simulink library "spikertlib"  (R2024b)
settings: Solver=FixedStepAuto  StartTime=0.0  StopTime=10.0  RelTol=1e-3
libraries: simulink x1, $bdroot x1
settings Model: Creator=ymatsuur  LastModifiedBy=yokano
settings OptimizationCC: DefaultParameterBehavior=Inlined  EnhancedBackFolding=on  PassReuseOutputArgsAs=Individual arguments  ZeroExternalMemoryAtStartup=off  ZeroInternalMemoryAtStartup=off  OptimizeBlockOrder=speed  DifferentSizesBufferReuse=on  OptimizationCustomize=off  EfficientTunableParamExpr=on
settings DebuggingCC: ParameterTunabilityLossMsg=error
settings SFSimCC: MATLABDynamicMemAlloc=off
settings RTWCC: Description=Embedded Coder  SystemTargetFile=ert.tlc  GenCodeOnly=on  TemplateMakefile=ert_default_tmf  GPUComputeCapability=3.5
settings CodeAppCC: ForceParamTrailComments=on  IgnoreCustomStorageClasses=off  OperatorAnnotations=on  SimulinkDataObjDesc=on  SFDataObjDesc=on  InsertBlockDesc=on
settings ERTTargetCC: TargetLangStandard=C99 (ISO)  GenerateSampleERTMain=on  IncludeMdlTerminateFcn=off  ERTCustomFileTemplate=addspikertmain.tlc  ERTFilePackagingFormat=Compact

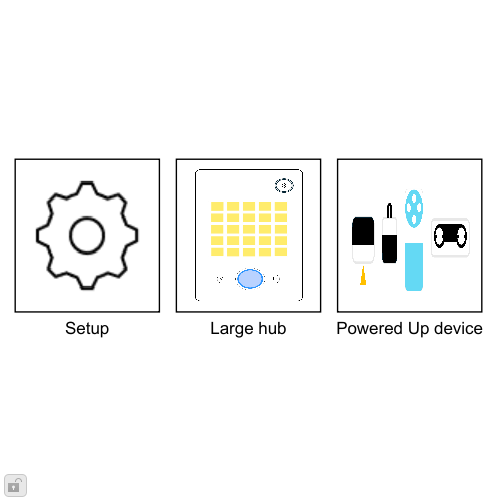
[thumbnail: Simulink's stored preview of the top-level diagram]
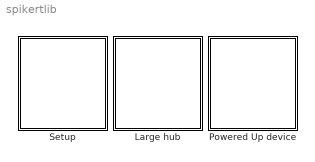
== system spikertlib ==
  Large hub : Subsystem
      mask Display: image('sphub.png'); % 変更するには、ツールストリップの [イメージの編集] を使用してください。
  Powered Up device : Subsystem
      mask Display: image('sppup.png'); % 変更するには、ツールストリップの [イメージの編集] を使用してください。
  Setup : Subsystem
      mask Display: image('spmodelsetup.png');

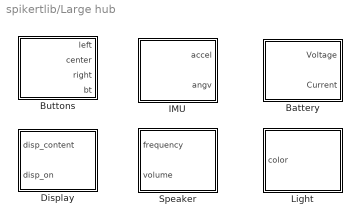
== system spikertlib/Large hub ==
  Battery : Subsystem  mask(Battery){}
      mask help: Retrieve the battery voltage [mV] and the battery current[mA].
      mask Display: image('spbattery.png');
  Buttons : Subsystem  mask(Buttons){}
      mask help: Checks which buttons (left, center, right, bluetooth) are currently pressed. (0=Not pressed, 1=Pressed)
      mask Display: image('spbutton.png');
  Display : Subsystem  mask(Pup device){Mode=Numeric, UpOrientation=RIGHT}
      mask prompts: UpOrientation "Upside orientation"
      mask help:
      | [Numeric]
      | Displays a number in the range -99 to 99. A minus sign (-) is shown as a faint dot in the center of the display. Upside orientation is set to TOP, LEFT, RIGHT, BOTTOM.
      |
      | [Character]
      | Display one character at a time if dispOn is greater than 0. Character input must be string type. Upside orientation is set to TOP, LEFT, RIGHT, BOTTOM.
      |
      | [Matrix]
      | Displays brightness matrix of Mux array in the range of 0-100. Upside orientation is set to TOP, LEFT, RIGHT, BOTTOM.
      mask TypeOptions Mode: Numeric | Character | Matrix
      mask TypeOptions UpOrientation: TOP | LEFT | RIGHT | BOTTOM
      mask DialogControl ParameterGroupVar Prompt: パラメーター
      mask Display: image('spdisplay.png');
  IMU : Subsystem  mask(Imu){}
      mask help:
      | Get the acceleration and angular velocity by the IMU.
      | accel: The vector signal which contains x, y, z axes of the acceleration [mm/s^2].
      | angv: The vector signal which contains x, y, z axes of the angular velocity [deg/sec].
      mask Display: image('spimu.png');
  Light : Subsystem  mask(Light){}
      mask help: Turn the light on with specified color (0=White, 1=Red, 2=Orange, 3=Yellow, 4=Green, 5=Blue, 6=Indigo, 7=Purple, Others=Off).
      mask Display: image('splight.png');
  Speaker : Subsystem  mask(Speaker){}
      mask help:
      | Set the volume level of the speaker and play a tone.
      | volume range 0-100[%], and frequency range 0-24000[Hz].
      mask Display: image('spspeaker.png');

== system spikertlib/Powered Up device ==
  PortA In : Subsystem  mask(Pup device){PortID=A, SensorType=Force, SensorMode=Reflection, LightOn=on}
      mask prompts: PortID "Port"; SensorType "Sensor type"; SensorMode "Sensor mode"; LightOn "Light on"
      mask help:
      | [Force sensor]
      | Force sensor detects the force [N] (range: about 0-10).
      |
      | [Color sensor]
      | Color sensor detect the reflection, ambient light, or color (HSV).
      | Reflection: Get the percentage of how much a surface reflects the light emitted by the sensor. [%] (100= white, 50= gray, 01=black, 00=No surface in front of the sensor.)
      | Ambient: Get the ambient light intensity (range: 0=dark, 100=bright)
      | Color: Get the color of surface. (0=Others, 1=Red, 2=Orange, 3=Yellow, 4=Green, 5=Blue, 6=Indigo, 7=Violet)
      |
      | [Ultrasonic sensor]
      | Get the distance [mm] in front of the ultrasonic sensor. (range: 0-2000, 2000 if no obstacles in front of the sensor.)
      |
      | [Motor]
      | Get the angle[deg] angle velocity [deg/s] of the motor.
      | !! Need Motor block in the same model for initialization. !!
      |
      | [None]
      | No sensor exsists.
      mask TypeOptions PortID: A | B | C | D | E | F
      mask Callback PortID:
      | outportHandle = get_param([gcb, '/Out1'], 'PortHandles');
      |     lineHandle = get_param(outportHandle.Inport, 'Line');
      |     set_param(lineHandle, 'Name', get_param(gcb, 'SensorType') +"_"+ get_param(gcb, 'PortID'));
      mask TypeOptions SensorType: Force | Color | Ultrasonic | Motor | None
      mask Callback SensorType:
      | if get_param(gcb, 'SensorType') == "Force"
      |         set_param(gcb, 'MaskVisibilities', {'on', 'on', 'off', 'off'});
      |     elseif get_param(gcb, 'SensorType') == "Color"
      |         set_param(gcb, 'MaskVisibilities', {'on', 'on', 'on', 'on'});
      |     elseif get_param(gcb, 'SensorType') == "Ultrasonic"
      |         set_param(gcb, 'MaskVisibilities', {'on', 'on', 'off', 'on'});
      |     else
      |         set_param(gcb, 'MaskVisibilities', {'on', 'on', 'off', 'off'});
      |     end
      | 
      |     outportHandle = get_param([gcb, '/Out1'], 'PortHandles');
      |     lineHandle = get_param(outportHandle.Inport, 'Line');
      |     set_param(lineHandle, 'Name', get_param(gcb, 'SensorType') +"_"+ get_param(gcb, 'PortID'));
      mask TypeOptions SensorMode: Reflection | Ambient | Color
      mask DialogControl ParameterGroupVar Prompt: パラメーター
      mask Display:
      | switch get_param(gcb, 'SensorType')
      |     case "Force"
      |         image('spforcesensor.png');
      |     case "Color"
      |         image('spcolorsensor.png');
      |     case "Ultrasonic"
      |         image('spultrasonicsensor.png');
      |     case "Motor"
      |         image('spmotor.png');
      |     case 5
      |         disp("");
      | end
      | 
      | color('red');
      | switch get_param(gcb, 'PortID')
      |     case "A"
      |         text(0.7, 0.1, 'Port: A');
      |     case "B"
      |         text(0.7, 0.1, 'Port: B');
      |     case "C"
      |         text(0.7, 0.1, 'Port: C');
      |     case "D"
      |         text(0.7, 0.1, 'Port: D');
      |     case "E"
      |         text(0.7, 0.1, 'Port: E');
      |     case "F"
      |         text(0.7, 0.1, 'Port: F');
      | end
  PortA Out : Subsystem  mask(Pup device){PortID=A, Mode=Set the speed of rotation [deg/s], EncorderReset=No reset, Direction=Clockwise}
      mask prompts: PortID "Port"; Mode "Motor mode"; EncorderReset "Encorder"
      mask help:
      | [Motor mode]
      | Set the speed of rotation[deg/s]: Control the motor speed at the specified value.
      | Set the power of the motor[%]: Set the motor voltage.
      | Stop: Stop the motor. But, the encoder is active and the value can be used.
      |
      | [Encorder]
      | No reset: Initial encorder value is set to an absolute angle.
      | Reset: Initial encorder value is set to 0.
      mask TypeOptions PortID: A | B | C | D | E | F
      mask Callback PortID:
      | outportHandle = get_param([gcb, '/In1'], 'PortHandles');
      |     lineHandle = get_param(outportHandle.Outport, 'Line');
      | 
      |     if get_param(gcb, 'Mode') == "None"
      |         set_param(gcb, 'MaskVisibilities', {'on', 'on', 'off', 'off'});
      |         set_param(lineHandle, 'Name', "Motor_"+ get_param(gcb, 'PortID'));
      |     else
      |         set_param(gcb, 'MaskVisibilities', {'on', 'on', 'on', 'on'});
      |         set_param(lineHandle, 'Name', "None_"+ get_param(gcb, 'PortID'));
      |     end
      mask Callback Mode:
      | outportHandle = get_param([gcb, '/In1'], 'PortHandles');
      |     lineHandle = get_param(outportHandle.Outport, 'Line');
      | 
      |     if get_param(gcb, 'Mode') == "None"
      |         set_param(gcb, 'MaskVisibilities', {'on', 'on', 'off', 'off'});
      |         set_param(lineHandle, 'Name', "Motor_"+ get_param(gcb, 'PortID'));
      |     else
      |         set_param(gcb, 'MaskVisibilities', {'on', 'on', 'on', 'on'});
      |         set_param(lineHandle, 'Name', "None_"+ get_param(gcb, 'PortID'));
      |     end
      mask TypeOptions EncorderReset: No reset | Reset
      mask TypeOptions Direction: Clockwise | Couter-clockwise
      mask DialogControl ParameterGroupVar Prompt: パラメーター
      mask Display:
      | if get_param(gcb, 'Mode') == "None"
      | 
      | else
      |     image('spmotor.png');
      | end
      | 
      | 
      | color('red');
      | switch get_param(gcb, 'PortID')
      |     case "A"
      |         text(0.7, 0.1, 'Port: A');
      |     case "B"
      |         text(0.7, 0.1, 'Port: B');
      |     case "C"
      |         text(0.7, 0.1, 'Port: C');
      |     case "D"
      |         text(0.7, 0.1, 'Port: D');
      |     case "E"
      |         text(0.7, 0.1, 'Port: E');
      |     case "F"
      |         text(0.7, 0.1, 'Port: F');
      | end

== system spikertlib/Setup ==
  Callback Button : CustomCallbackButton  Description=Generate and build code. write executable to SPIKE  Configuration="{\"components\":[{\"name\":\"BackgroundImageComponent\",\"settings\":{\"image\":{\"size\":[0,0],\"src\":\"default\",\"srcOrientation\":\"Right\"},\"position\":[0,0,1,1]}},{\"name\":\"ButtonStateComponent\",\"settings\":{\"buttonType\":\"momentary\",\"clickFcn\":\"controlsetupspikert_callback;\\ncopyspikert(2)\\ncopyspikert(3)\",\"latched\":false,\"offValue\":null,\"onValue\":1,\"position\":[0,0,1,1],\"pressDelay\":\"500\",\"pressFcn\":\"\",\"repeatInterval\":\"0\",\"states\":[{\"horizontalAlignment\":\"center\",\"image\":{\"position\":[0,0,1,1],\"size\":[1,1],\"src\":\"default\",\"srcOrientation\":\"Right\"},\"label\":{\"color\":[1,1,1],\"icon\":{\"size\":[0,0],\"src\":\"default\",\"srcOrientation\":\"Right\"},\"iconOffset\":0,\"iconPlacement\":\"left\",\"opacity\":1,\"show\":true,\"text\":{\"content\":\"Build & Write\",\"font\":\"Helvetica\"}},\"labelOffset\":[0,0],\"verticalAlignment\":\"middle\"},{\"horizontalAlignment\":\"center\",\"image\":{\"position\":[0,0,1,1],\"size\":[1,1],\"src\":\"default\",\"srcOrientation\":\"Right\"},\"label\":{\"color\":[0.01176470588,0.01176470588,0.01176470588,1],\"icon\":{\"size\":[0,0],\"src\":\"default\",\"srcOrientation\":\"Right\"},\"iconOffset\":0,\"iconPlacement\":\"left\",\"opacity\":1,\"show\":true,\"text\":{\"content\":\"Build & Write\",\"font\":\"Helvetica\"}},\"labelOffset\":[0,0],\"verticalAlignment\":\"middle\"},{\"horizontalAlignment\":\"center\",\"image\":{\"position\":[0,0,1,1],\"size\":[1,1],\"src\":\"default\",\"srcOrientation\":\"Right\"},\"label\":{\"color\":[0.01176470588,0.01176470588,0.01176470588,1],\"icon\":{\"size\":[0,0],\"src\":\"default\",\"srcOrientation\":\"Right\"},\"iconOffset\":0,\"iconPlacement\":\"left\",\"opacity\":1,\"show\":true,\"text\":{\"content\":\"Build & Write\",\"font\":\"Helvetica\"}},\"labelOffset\":[0,0],\"verticalAlignment\":\"middle\"},{\"horizontalAlignment\":\"center\",\"image\":{\"position\":[0,0,1,1],\"size\":[1,1],\"src\":\"default\",\"srcOrientation\":\"Right\"},\"label\":{\"color\":[0.01176470588,0.01176470588,0.01176470588,1],\"icon\":{\"size\":[0,0],\"src\":\"default\",\"srcOrientation\":\"Right\"},\"iconOffset\":0,\"iconPlacement\":\"left\",\"opacity\":1,\"show\":true,\"text\":{\"content\":\"Build & Write\",\"font\":\"Helvetica\"}},\"labelOffset\":[0,0],\"verticalAlignment\":\"middle\"}]}},{\"name\":\"ForegroundImageComponent\",\"settings\":{\"image\":{\"size\":[0,0],\"src\":\"default\",\"srcOrientation\":\"Right\"},\"isForeground\":1,\"position\":[0,0,1,1]}}],\"settings\":{\"BindingType\":\"standalone\",\"backgroundColor\":[244,244,244,1],\"backgroundOffset\":0.2,\"backgroundOpacity\":1,\"fixedAspectRatio\":\"off\",\"foregroundColor\":[0.01176470588,0.01176470588,0.01176470588,1],\"migratedFromLegacy\":true,\"useBackgroundColor\":true,\"variant\":\"callback\",\"version\":\"R2023a\"},\"type\":\"Button\"}"  CustomBackgroundColor="{\"color\":[0.8509803921568627,0.3254901960784314,0.09803921568627451],\"show\":true}"
  Callback Button1 : CustomCallbackButton  Description=Generate and build code. write executable to SPIKE  Configuration="{\"components\":[{\"name\":\"BackgroundImageComponent\",\"settings\":{\"image\":{\"size\":[0,0],\"src\":\"default\",\"srcOrientation\":\"Right\"},\"position\":[0,0,1,1]}},{\"name\":\"ButtonStateComponent\",\"settings\":{\"buttonType\":\"momentary\",\"clickFcn\":\"copyspikert(4)\",\"latched\":false,\"offValue\":null,\"onValue\":1,\"position\":[0,0,1,1],\"pressDelay\":\"500\",\"pressFcn\":\"\",\"repeatInterval\":\"0\",\"states\":[{\"horizontalAlignment\":\"center\",\"image\":{\"position\":[0,0,1,1],\"size\":[1,1],\"src\":\"default\",\"srcOrientation\":\"Right\"},\"label\":{\"color\":[1,1,1],\"icon\":{\"size\":[0,0],\"src\":\"default\",\"srcOrientation\":\"Right\"},\"iconOffset\":0,\"iconPlacement\":\"left\",\"opacity\":1,\"show\":true,\"text\":{\"content\":\"Restore original firmware\",\"font\":\"Helvetica\"}},\"labelOffset\":[0,0],\"verticalAlignment\":\"middle\"},{\"horizontalAlignment\":\"center\",\"image\":{\"position\":[0,0,1,1],\"size\":[1,1],\"src\":\"default\",\"srcOrientation\":\"Right\"},\"label\":{\"color\":[0.01176470588,0.01176470588,0.01176470588,1],\"icon\":{\"size\":[0,0],\"src\":\"default\",\"srcOrientation\":\"Right\"},\"iconOffset\":0,\"iconPlacement\":\"left\",\"opacity\":1,\"show\":true,\"text\":{\"content\":\"Restore original firmware\",\"font\":\"Helvetica\"}},\"labelOffset\":[0,0],\"verticalAlignment\":\"middle\"},{\"horizontalAlignment\":\"center\",\"image\":{\"position\":[0,0,1,1],\"size\":[1,1],\"src\":\"default\",\"srcOrientation\":\"Right\"},\"label\":{\"color\":[0.01176470588,0.01176470588,0.01176470588,1],\"icon\":{\"size\":[0,0],\"src\":\"default\",\"srcOrientation\":\"Right\"},\"iconOffset\":0,\"iconPlacement\":\"left\",\"opacity\":1,\"show\":true,\"text\":{\"content\":\"Restore original firmware\",\"font\":\"Helvetica\"}},\"labelOffset\":[0,0],\"verticalAlignment\":\"middle\"},{\"horizontalAlignment\":\"center\",\"image\":{\"position\":[0,0,1,1],\"size\":[1,1],\"src\":\"default\",\"srcOrientation\":\"Right\"},\"label\":{\"color\":[0.01176470588,0.01176470588,0.01176470588,1],\"icon\":{\"size\":[0,0],\"src\":\"default\",\"srcOrientation\":\"Right\"},\"iconOffset\":0,\"iconPlacement\":\"left\",\"opacity\":1,\"show\":true,\"text\":{\"content\":\"Restore original firmware\",\"font\":\"Helvetica\"}},\"labelOffset\":[0,0],\"verticalAlignment\":\"middle\"}]}},{\"name\":\"ForegroundImageComponent\",\"settings\":{\"image\":{\"size\":[0,0],\"src\":\"default\",\"srcOrientation\":\"Right\"},\"isForeground\":1,\"position\":[0,0,1,1]}}],\"settings\":{\"BindingType\":\"standalone\",\"backgroundColor\":[244,244,244,1],\"backgroundOffset\":0.2,\"backgroundOpacity\":1,\"fixedAspectRatio\":\"off\",\"foregroundColor\":[0.01176470588,0.01176470588,0.01176470588,1],\"migratedFromLegacy\":true,\"useBackgroundColor\":true,\"variant\":\"callback\",\"version\":\"R2023a\"},\"type\":\"Button\"}"  CustomBackgroundColor="{\"color\":[0,0.4470588235294118,0.7411764705882353],\"show\":true}"

== system spikertlib/Large hub/Battery ==
  Battery : S-Function  FunctionName=Battery  SFunctionDeploymentMode=off  EnableBusSupport=off  mask(Legacy Function){SFunctionSpec=Battery(double y1, double y2), ShowSpec=on}
      mask prompts: ShowSpec "表示関数の仕様"
      mask help:
      | このブロックは、以下の Legacy Code Tool の定義で指定されたレガシ関数を呼び出すことができます:
      | def.SFunctionName = 'Battery';
      | def.OutputFcnSpec = 'Battery(double y1, double y2)';
      | def.HeaderFiles = {'sfunspikert.h'};
      | def.SourceFiles = {'sfunspikert.c'};
      | def.IncPaths = {'C:\class\coursefiles\SPIKE_Dev\libblocks'};
      mask Help: <p>このブロックは、Legacy Code Tool で自動的に生成されました。このツールと呼び出しの詳細は、ヘルプを参照してください。<a href="matlab:legacy_code('help')"> legacy_code('help')</a>.</p>
      mask Callback ShowSpec:
      | if strcmp(get_param(gcbh, 'ShowSpec'), 'on')
      |   set_param(gcbh, 'MaskDisplay', sprintf('fprintf(''%s'');', get_param(gcbh, 'SFunctionSpec')));
      | else
      |   set_param(gcbh, 'MaskDisplay', sprintf('fprintf(''%s'');', get_param(gcbh, 'FunctionName')));
      | end
      mask Display: fprintf('Battery(double y1, double y2)');
  Voltage : Outport
  Current : Outport  Port=2
  wires:
  Battery/1 -> Voltage/1
  Battery/2 -> Current/1

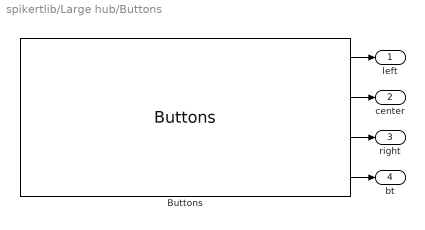
== system spikertlib/Large hub/Buttons ==
  Buttons : S-Function  FunctionName=Buttons  SFunctionDeploymentMode=off  EnableBusSupport=off  mask(Legacy Function){SFunctionSpec=Buttons(double y1[1], double y2[1], double y3[1], double y4[1]), ShowSpec=on}
      mask prompts: ShowSpec "表示関数の仕様"
      mask help:
      | このブロックは、以下の Legacy Code Tool の定義で指定されたレガシ関数を呼び出すことができます:
      | def.SFunctionName = 'Buttons';
      | def.OutputFcnSpec = 'Buttons(double y1[1], double y2[1], double y3[1], double y4[1])';
      | def.HeaderFiles = {'sfunspikert.h'};
      | def.SourceFiles = {'sfunspikert.c'};
      | def.IncPaths = {'C:\class\coursefiles\spikertlib\libblocks'};
      mask Help: <p>このブロックは、Legacy Code Tool で自動的に生成されました。このツールと呼び出しの詳細は、ヘルプを参照してください。<a href="matlab:legacy_code('help')"> legacy_code('help')</a>.</p>
      mask Callback ShowSpec:
      | if strcmp(get_param(gcbh, 'ShowSpec'), 'on')
      |   set_param(gcbh, 'MaskDisplay', sprintf('fprintf(''%s'');', get_param(gcbh, 'SFunctionSpec')));
      | else
      |   set_param(gcbh, 'MaskDisplay', sprintf('fprintf(''%s'');', get_param(gcbh, 'FunctionName')));
      | end
      mask Display: fprintf('Buttons(double y1[1], double y2[1], double y3[1], double y4[1])');
  left : Outport
  center : Outport  Port=2
  right : Outport  Port=3
  bt : Outport  Port=4
  wires:
  Buttons/1 -> left/1
  Buttons/2 -> center/1
  Buttons/3 -> right/1
  Buttons/4 -> bt/1

== system spikertlib/Large hub/Display ==
  disp_content : Inport
  disp_on : Inport  Port=2
  Subsystem : Subsystem  Variant=on  VariantControl=Subsystem
  wires:
  disp_on/1 -> Subsystem/2(disp_on)
  disp_content/1 -> Subsystem/1(disp_content)

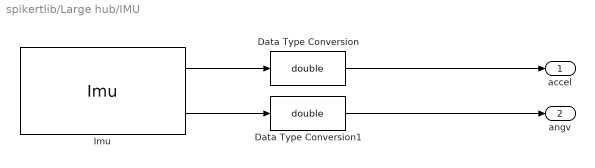
== system spikertlib/Large hub/IMU ==
  Data Type Conversion : DataTypeConversion  OutDataTypeStr=double  SaturateOnIntegerOverflow=off  RndMeth=Floor
  Data Type Conversion1 : DataTypeConversion  OutDataTypeStr=double  SaturateOnIntegerOverflow=off  RndMeth=Floor
  Imu : S-Function  FunctionName=Imu  SFunctionDeploymentMode=off  EnableBusSupport=off  mask(Legacy Function){SFunctionSpec=Imu(single y1[3], single y2[3]), ShowSpec=on}
      mask prompts: ShowSpec "表示関数の仕様"
      mask help:
      | このブロックは、以下の Legacy Code Tool の定義で指定されたレガシ関数を呼び出すことができます:
      | def.SFunctionName = 'Imu';
      | def.OutputFcnSpec = 'Imu(single y1[3], single y2[3])';
      | def.StartFcnSpec = 'ImuInit()';
      | def.HeaderFiles = {'sfunspikert.h'};
      | def.SourceFiles = {'sfunspikert.c'};
      | def.IncPaths = {'C:\class\coursefiles\spikertlib\libblocks'};
      mask Help: <p>このブロックは、Legacy Code Tool で自動的に生成されました。このツールと呼び出しの詳細は、ヘルプを参照してください。<a href="matlab:legacy_code('help')"> legacy_code('help')</a>.</p>
      mask Callback ShowSpec:
      | if strcmp(get_param(gcbh, 'ShowSpec'), 'on')
      |   set_param(gcbh, 'MaskDisplay', sprintf('fprintf(''%s'');', get_param(gcbh, 'SFunctionSpec')));
      | else
      |   set_param(gcbh, 'MaskDisplay', sprintf('fprintf(''%s'');', get_param(gcbh, 'FunctionName')));
      | end
      mask Display: fprintf('Imu(single y1[3], single y2[3])');
  accel : Outport
  angv : Outport  Port=2
  wires:
  Data Type Conversion/1 -> accel/1
  Data Type Conversion1/1 -> angv/1
  Imu/2 -> Data Type Conversion1/1
  Imu/1 -> Data Type Conversion/1

== system spikertlib/Large hub/Light ==
  color : Inport
  Light : S-Function  FunctionName=Light  SFunctionDeploymentMode=off  EnableBusSupport=off  mask(Legacy Function){SFunctionSpec=Light(double u1), ShowSpec=on}
      mask prompts: ShowSpec "表示関数の仕様"
      mask help:
      | このブロックは、以下の Legacy Code Tool の定義で指定されたレガシ関数を呼び出すことができます:
      | def.SFunctionName = 'Light';
      | def.OutputFcnSpec = 'Light(double u1)';
      | def.StartFcnSpec = 'LightInit()';
      | def.HeaderFiles = {'sfunspikert.h'};
      | def.SourceFiles = {'sfunspikert.c'};
      | def.IncPaths = {'C:\class\coursefiles\spikertlib\libblocks'};
      mask Help: <p>このブロックは、Legacy Code Tool で自動的に生成されました。このツールと呼び出しの詳細は、ヘルプを参照してください。<a href="matlab:legacy_code('help')"> legacy_code('help')</a>.</p>
      mask Callback ShowSpec:
      | if strcmp(get_param(gcbh, 'ShowSpec'), 'on')
      |   set_param(gcbh, 'MaskDisplay', sprintf('fprintf(''%s'');', get_param(gcbh, 'SFunctionSpec')));
      | else
      |   set_param(gcbh, 'MaskDisplay', sprintf('fprintf(''%s'');', get_param(gcbh, 'FunctionName')));
      | end
      mask Display: fprintf('Light(double u1)');
  wires:
  color/1 -> Light/1

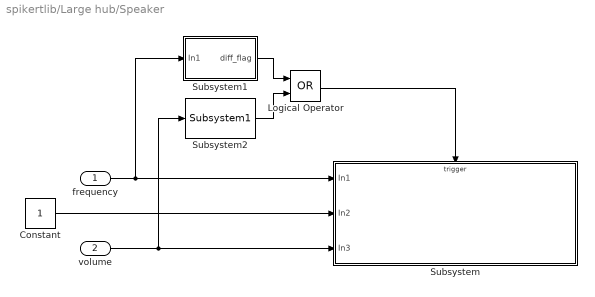
== system spikertlib/Large hub/Speaker ==
  frequency : Inport
  volume : Inport  Port=2
  Constant : Constant
  Logical Operator : Logic  Operator=OR  AllPortsSameDT=off  OutDataTypeStr=boolean
  Subsystem : Subsystem
  Subsystem1 : Subsystem
  Subsystem2 : $bdroot/Large hub/Speaker/Subsystem1  SystemSampleTime=-1  VariantActivationTime=update diagram  AllowFlexibleInterface=on  Latency=0  AutoFrameSizeCalculation=off
  wires:
  frequency/1 -> Subsystem1/1(In1), Subsystem/1(In1)
  Constant/1 -> Subsystem/2(In2)
  volume/1 -> Subsystem2/1, Subsystem/3(In3)
  Subsystem1/1(diff_flag) -> Logical Operator/1
  Subsystem2/1 -> Logical Operator/2
  Logical Operator/1 -> Subsystem/Trigger

== system spikertlib/Powered Up device/PortA In ==
  Subsystem : Subsystem  Variant=on  VariantControl=Subsystem
  Out1 : Outport
  wires:
  Subsystem/1(Out1) -> Out1/1  "Force_A"

== system spikertlib/Powered Up device/PortA Out ==
  In1 : Inport
  Subsystem : Subsystem  Variant=on  VariantControl=Subsystem
  wires:
  In1/1 -> Subsystem/1(In1)  "None_A"

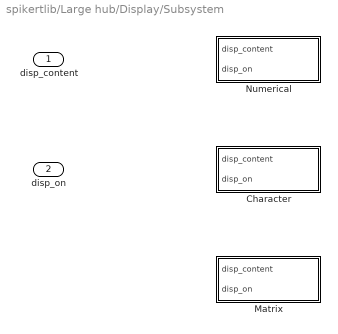
== system spikertlib/Large hub/Display/Subsystem ==
  disp_content : Inport
  disp_on : Inport  Port=2
  Character : Subsystem  VariantControl=Mode==2
  Matrix : Subsystem  VariantControl=Mode==3
  Numerical : Subsystem  VariantControl=Mode==1

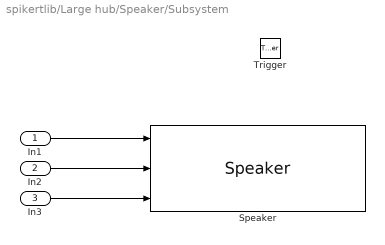
== system spikertlib/Large hub/Speaker/Subsystem ==
  In1 : Inport
  In2 : Inport  Port=2
  In3 : Inport  Port=3
  Trigger : TriggerPort  VariantControl=(inherit)  PortDimensions=1
  Speaker : S-Function  FunctionName=Speaker  SFunctionDeploymentMode=off  EnableBusSupport=off  mask(Legacy Function){SFunctionSpec=Speaker(double u1, double u2, double u3), ShowSpec=on}
      mask prompts: ShowSpec "表示関数の仕様"
      mask help:
      | このブロックは、以下の Legacy Code Tool の定義で指定されたレガシ関数を呼び出すことができます:
      | def.SFunctionName = 'Speaker';
      | def.OutputFcnSpec = 'Speaker(double u1, double u2, double u3)';
      | def.HeaderFiles = {'sfunspikert.h'};
      | def.SourceFiles = {'sfunspikert.c'};
      | def.IncPaths = {'C:\class\coursefiles\spikertlib\libblocks'};
      mask Help: <p>このブロックは、Legacy Code Tool で自動的に生成されました。このツールと呼び出しの詳細は、ヘルプを参照してください。<a href="matlab:legacy_code('help')"> legacy_code('help')</a>.</p>
      mask Callback ShowSpec:
      | if strcmp(get_param(gcbh, 'ShowSpec'), 'on')
      |   set_param(gcbh, 'MaskDisplay', sprintf('fprintf(''%s'');', get_param(gcbh, 'SFunctionSpec')));
      | else
      |   set_param(gcbh, 'MaskDisplay', sprintf('fprintf(''%s'');', get_param(gcbh, 'FunctionName')));
      | end
      mask Display: fprintf('Speaker(double u1, double u2, double u3)');
  wires:
  In3/1 -> Speaker/3
  In2/1 -> Speaker/2
  In1/1 -> Speaker/1

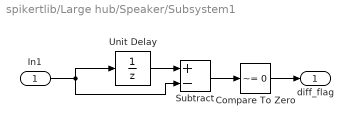
== system spikertlib/Large hub/Speaker/Subsystem1 ==
  In1 : Inport
  Compare To Zero : simulink/Logic and Bit Operations/Compare To Zero  relop=~=  OutDataTypeStr=boolean
  Subtract : Sum  Inputs=+-
  Unit Delay : UnitDelay  SampleTime=-1  HasFrameUpgradeWarning=on
  diff_flag : Outport
  wires:
  In1/1 -> Subtract/2, Unit Delay/1
  Unit Delay/1 -> Subtract/1
  Subtract/1 -> Compare To Zero/1
  Compare To Zero/1 -> diff_flag/1

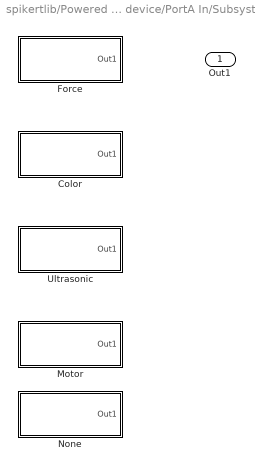
== system spikertlib/Powered Up device/PortA In/Subsystem ==
  Color : Subsystem  VariantControl=SensorType==2
  Force : Subsystem  VariantControl=SensorType==1
  Motor : Subsystem  VariantControl=SensorType==4
  None : Subsystem  VariantControl=SensorType==5
  Ultrasonic : Subsystem  VariantControl=SensorType==3
  Out1 : Outport

== system spikertlib/Powered Up device/PortA Out/Subsystem ==
  In1 : Inport
  Motor : Subsystem  VariantControl=Mode~=4
  None : Subsystem  VariantControl=Mode==4

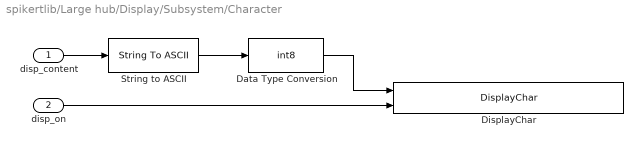
== system spikertlib/Large hub/Display/Subsystem/Character ==
  disp_content : Inport
  disp_on : Inport  Port=2
  Data Type Conversion : DataTypeConversion  OutDataTypeStr=int8  SaturateOnIntegerOverflow=off  RndMeth=Floor
  DisplayChar : S-Function  FunctionName=DisplayChar  Parameters=SParameter1  SFunctionDeploymentMode=off  EnableBusSupport=off  mask(Legacy Function){SFunctionSpec=Displaychar(int8 u1, double u2, double p1), SParameter1=UpOrientation-1, ShowSpec=on}
      mask prompts: SParameter1 "P1:"; ShowSpec "表示関数の仕様"
      mask help:
      | このブロックは、以下の Legacy Code Tool の定義で指定されたレガシ関数を呼び出すことができます:
      | def.SFunctionName = 'DisplayChar';
      | def.OutputFcnSpec = 'Displaychar(int8 u1, double u2, double p1)';
      | def.StartFcnSpec = 'DisplaycharInit()';
      | def.HeaderFiles = {'sfunspikert.h'};
      | def.SourceFiles = {'sfunspikert.c'};
      | def.IncPaths = {'C:\class\coursefiles\SPIKE_Dev\libblocks'};
      mask Help: <p>このブロックは、Legacy Code Tool で自動的に生成されました。このツールと呼び出しの詳細は、ヘルプを参照してください。<a href="matlab:legacy_code('help')"> legacy_code('help')</a>.</p>
      mask Callback ShowSpec:
      | if strcmp(get_param(gcbh, 'ShowSpec'), 'on')
      |   set_param(gcbh, 'MaskDisplay', sprintf('fprintf(''%s'');', get_param(gcbh, 'SFunctionSpec')));
      | else
      |   set_param(gcbh, 'MaskDisplay', sprintf('fprintf(''%s'');', get_param(gcbh, 'FunctionName')));
      | end
      mask Display: fprintf('Displaychar(int8 u1, double u2, double p1)');
  String to ASCII : StringToASCII  OutputVectorSize=1
  wires:
  disp_content/1 -> String to ASCII/1
  String to ASCII/1 -> Data Type Conversion/1
  Data Type Conversion/1 -> DisplayChar/1
  disp_on/1 -> DisplayChar/2

== system spikertlib/Large hub/Display/Subsystem/Matrix ==
  disp_content : Inport
  disp_on : Inport  Port=2
  DisplayMatrix1 : S-Function  FunctionName=DisplayMatrix  Parameters=SParameter1  SFunctionDeploymentMode=off  EnableBusSupport=off  mask(Legacy Function){SFunctionSpec=Displaymat(double u1[25], double u2, double p1), SParameter1=UpOrientation-1, ShowSpec=on}
      mask prompts: SParameter1 "P1:"; ShowSpec "表示関数の仕様"
      mask help:
      | このブロックは、以下の Legacy Code Tool の定義で指定されたレガシ関数を呼び出すことができます:
      | def.SFunctionName = 'DisplayMatrix';
      | def.OutputFcnSpec = 'Displaymat(double u1[25], double u2, double p1)';
      | def.StartFcnSpec = 'DisplaymatInit()';
      | def.HeaderFiles = {'sfunspikert.h'};
      | def.SourceFiles = {'sfunspikert.c'};
      | def.IncPaths = {'C:\class\coursefiles\spikertlib\libblocks'};
      mask Help: <p>このブロックは、Legacy Code Tool で自動的に生成されました。このツールと呼び出しの詳細は、ヘルプを参照してください。<a href="matlab:legacy_code('help')"> legacy_code('help')</a>.</p>
      mask Callback ShowSpec:
      | if strcmp(get_param(gcbh, 'ShowSpec'), 'on')
      |   set_param(gcbh, 'MaskDisplay', sprintf('fprintf(''%s'');', get_param(gcbh, 'SFunctionSpec')));
      | else
      |   set_param(gcbh, 'MaskDisplay', sprintf('fprintf(''%s'');', get_param(gcbh, 'FunctionName')));
      | end
      mask Display: fprintf('Displaymat(double u1[25], double u2, double p1)');
  wires:
  disp_on/1 -> DisplayMatrix1/2
  disp_content/1 -> DisplayMatrix1/1

== system spikertlib/Large hub/Display/Subsystem/Numerical ==
  disp_content : Inport
  disp_on : Inport  Port=2
  DisplayNumber1 : S-Function  FunctionName=DisplayNumber  Parameters=SParameter1  SFunctionDeploymentMode=off  EnableBusSupport=off  mask(Legacy Function){SFunctionSpec=Displaynum(double u1, double u2, double p1), SParameter1=UpOrientation-1, ShowSpec=on}
      mask prompts: SParameter1 "P1:"; ShowSpec "表示関数の仕様"
      mask help:
      | このブロックは、以下の Legacy Code Tool の定義で指定されたレガシ関数を呼び出すことができます:
      | def.SFunctionName = 'DisplayNumber';
      | def.OutputFcnSpec = 'Displaynum(double u1, double u2, double p1)';
      | def.StartFcnSpec = 'DisplaynumInit()';
      | def.HeaderFiles = {'sfunspikert.h'};
      | def.SourceFiles = {'sfunspikert.c'};
      | def.IncPaths = {'C:\class\coursefiles\spikertlib\libblocks'};
      mask Help: <p>このブロックは、Legacy Code Tool で自動的に生成されました。このツールと呼び出しの詳細は、ヘルプを参照してください。<a href="matlab:legacy_code('help')"> legacy_code('help')</a>.</p>
      mask Callback ShowSpec:
      | if strcmp(get_param(gcbh, 'ShowSpec'), 'on')
      |   set_param(gcbh, 'MaskDisplay', sprintf('fprintf(''%s'');', get_param(gcbh, 'SFunctionSpec')));
      | else
      |   set_param(gcbh, 'MaskDisplay', sprintf('fprintf(''%s'');', get_param(gcbh, 'FunctionName')));
      | end
      mask Display: fprintf('Displaynum(double u1, double u2, double p1)');
  wires:
  disp_content/1 -> DisplayNumber1/1
  disp_on/1 -> DisplayNumber1/2

== system spikertlib/Powered Up device/PortA In/Subsystem/Color ==
  Colorsensor1 : S-Function  FunctionName=Colorsensor  Parameters=SParameter1, SParameter2, SParameter3  SFunctionDeploymentMode=off  EnableBusSupport=off  mask(Legacy Function){SFunctionSpec=double y1 = Colorsensor(double p1, double p2, double p3), SParameter1=PortID-1, SParameter2=SensorMode-1, SParameter3=LightOn, ShowSpec=on}
      mask prompts: SParameter1 "P1:"; SParameter2 "P2:"; SParameter3 "P3:"; ShowSpec "表示関数の仕様"
      mask help:
      | このブロックは、以下の Legacy Code Tool の定義で指定されたレガシ関数を呼び出すことができます:
      | def.SFunctionName = 'Colorsensor';
      | def.OutputFcnSpec = 'double y1 = Colorsensor(double p1, double p2, double p3)';
      | def.StartFcnSpec = 'ColorsensorInit()';
      | def.HeaderFiles = {'sfunspikert.h'};
      | def.SourceFiles = {'sfunspikert.c'};
      | def.IncPaths = {'C:\class\coursefiles\spikertlib\libblocks'};
      mask Help: <p>このブロックは、Legacy Code Tool で自動的に生成されました。このツールと呼び出しの詳細は、ヘルプを参照してください。<a href="matlab:legacy_code('help')"> legacy_code('help')</a>.</p>
      mask Callback ShowSpec:
      | if strcmp(get_param(gcbh, 'ShowSpec'), 'on')
      |   set_param(gcbh, 'MaskDisplay', sprintf('fprintf(''%s'');', get_param(gcbh, 'SFunctionSpec')));
      | else
      |   set_param(gcbh, 'MaskDisplay', sprintf('fprintf(''%s'');', get_param(gcbh, 'FunctionName')));
      | end
      mask Display: fprintf('double y1 = Colorsensor(double p1, double p2, double p3)');
  Out1 : Outport
  wires:
  Colorsensor1/1 -> Out1/1

== system spikertlib/Powered Up device/PortA In/Subsystem/Force ==
  Forcesensor1 : S-Function  FunctionName=Forcesensor  Parameters=SParameter1  SFunctionDeploymentMode=off  EnableBusSupport=off  mask(Legacy Function){SFunctionSpec=Forcesensor(double p1, double y1[1], double y2[1]), SParameter1=PortID-1, ShowSpec=on}
      mask prompts: SParameter1 "P1:"; ShowSpec "表示関数の仕様"
      mask help:
      | このブロックは、以下の Legacy Code Tool の定義で指定されたレガシ関数を呼び出すことができます:
      | def.SFunctionName = 'Forcesensor';
      | def.OutputFcnSpec = 'Forcesensor(double p1, double y1[1], double y2[1])';
      | def.StartFcnSpec = 'ForcesensorInit()';
      | def.HeaderFiles = {'sfunspikert.h'};
      | def.SourceFiles = {'sfunspikert.c'};
      | def.IncPaths = {'C:\class\coursefiles\spikertlib\libblocks'};
      mask Help: <p>このブロックは、Legacy Code Tool で自動的に生成されました。このツールと呼び出しの詳細は、ヘルプを参照してください。<a href="matlab:legacy_code('help')"> legacy_code('help')</a>.</p>
      mask Callback ShowSpec:
      | if strcmp(get_param(gcbh, 'ShowSpec'), 'on')
      |   set_param(gcbh, 'MaskDisplay', sprintf('fprintf(''%s'');', get_param(gcbh, 'SFunctionSpec')));
      | else
      |   set_param(gcbh, 'MaskDisplay', sprintf('fprintf(''%s'');', get_param(gcbh, 'FunctionName')));
      | end
      mask Display: fprintf('Forcesensor(double p1, double y1[1], double y2[1])');
  Terminator : Terminator
  Out1 : Outport
  wires:
  Forcesensor1/2 -> Terminator/1
  Forcesensor1/1 -> Out1/1

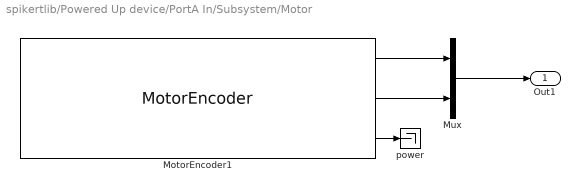
== system spikertlib/Powered Up device/PortA In/Subsystem/Motor ==
  MotorEncoder1 : S-Function  FunctionName=MotorEncoder  Parameters=SParameter1  SFunctionDeploymentMode=off  EnableBusSupport=off  mask(Legacy Function){SFunctionSpec=MotorEncoder(double p1, double y1[1], double y2[1], double y3[1]), SParameter1=PortID-1, ShowSpec=on}
      mask prompts: SParameter1 "P1:"; ShowSpec "表示関数の仕様"
      mask help:
      | このブロックは、以下の Legacy Code Tool の定義で指定されたレガシ関数を呼び出すことができます:
      | def.SFunctionName = 'MotorEncoder';
      | def.OutputFcnSpec = 'MotorEncoder(double p1, double y1[1], double y2[1], double y3[1])';
      | def.StartFcnSpec = 'MotorEncoderInit()';
      | def.HeaderFiles = {'sfunspikert.h'};
      | def.SourceFiles = {'sfunspikert.c'};
      | def.IncPaths = {'C:\class\coursefiles\spikertlib\libblocks'};
      mask Help: <p>このブロックは、Legacy Code Tool で自動的に生成されました。このツールと呼び出しの詳細は、ヘルプを参照してください。<a href="matlab:legacy_code('help')"> legacy_code('help')</a>.</p>
      mask Callback ShowSpec:
      | if strcmp(get_param(gcbh, 'ShowSpec'), 'on')
      |   set_param(gcbh, 'MaskDisplay', sprintf('fprintf(''%s'');', get_param(gcbh, 'SFunctionSpec')));
      | else
      |   set_param(gcbh, 'MaskDisplay', sprintf('fprintf(''%s'');', get_param(gcbh, 'FunctionName')));
      | end
      mask Display: fprintf('MotorEncoder(double p1, double y1[1], double y2[1], double y3[1])');
  Mux : Mux  Inputs=2
  power : Terminator
  Out1 : Outport
  wires:
  MotorEncoder1/3 -> power/1
  MotorEncoder1/1 -> Mux/1
  Mux/1 -> Out1/1
  MotorEncoder1/2 -> Mux/2

== system spikertlib/Powered Up device/PortA In/Subsystem/None ==
  Constant : Constant  Value=0
  Out1 : Outport
  wires:
  Constant/1 -> Out1/1

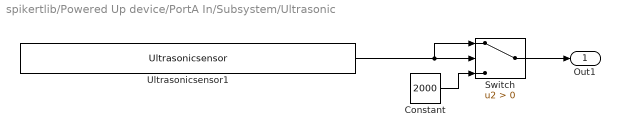
== system spikertlib/Powered Up device/PortA In/Subsystem/Ultrasonic ==
  Constant : Constant  Value=2000
  Switch : Switch  Criteria=u2 > Threshold  SaturateOnIntegerOverflow=off  InputSameDT=off
  Ultrasonicsensor1 : S-Function  FunctionName=Ultrasonicsensor  Parameters=SParameter1, SParameter2, SParameter3  SFunctionDeploymentMode=off  EnableBusSupport=off  mask(Legacy Function){SFunctionSpec=double y1 = Ultrasonicsensor(double p1, double p2, double p3), SParameter1=PortID-1, SParameter2=0, SParameter3=LightOn, ShowSpec=on}
      mask prompts: SParameter1 "P1:"; SParameter2 "P2:"; SParameter3 "P3:"; ShowSpec "表示関数の仕様"
      mask help:
      | このブロックは、以下の Legacy Code Tool の定義で指定されたレガシ関数を呼び出すことができます:
      | def.SFunctionName = 'Ultrasonicsensor';
      | def.OutputFcnSpec = 'double y1 = Ultrasonicsensor(double p1, double p2, double p3)';
      | def.StartFcnSpec = 'UltrasonicsensorInit()';
      | def.HeaderFiles = {'sfunspikert.h'};
      | def.SourceFiles = {'sfunspikert.c'};
      | def.IncPaths = {'C:\class\coursefiles\spikertlib\libblocks'};
      mask Help: <p>このブロックは、Legacy Code Tool で自動的に生成されました。このツールと呼び出しの詳細は、ヘルプを参照してください。<a href="matlab:legacy_code('help')"> legacy_code('help')</a>.</p>
      mask Callback ShowSpec:
      | if strcmp(get_param(gcbh, 'ShowSpec'), 'on')
      |   set_param(gcbh, 'MaskDisplay', sprintf('fprintf(''%s'');', get_param(gcbh, 'SFunctionSpec')));
      | else
      |   set_param(gcbh, 'MaskDisplay', sprintf('fprintf(''%s'');', get_param(gcbh, 'FunctionName')));
      | end
      mask Display: fprintf('double y1 = Ultrasonicsensor(double p1, double p2, double p3)');
  Out1 : Outport
  wires:
  Ultrasonicsensor1/1 -> Switch/1, Switch/2
  Switch/1 -> Out1/1
  Constant/1 -> Switch/3

== system spikertlib/Powered Up device/PortA Out/Subsystem/Motor ==
  In1 : Inport
  Motor2 : S-Function  FunctionName=Motor  Parameters=SParameter1, SParameter2, SParameter3, SParameter4  SFunctionDeploymentMode=off  EnableBusSupport=off  mask(Legacy Function){SFunctionSpec=Motor(double p1, double p2, double p3, double p4, double u1), SParameter1=PortID-1, SParameter2=Mode-1, SParameter3=EncorderReset -1, SParameter4=Direction -1, ShowSpec=on}
      mask prompts: SParameter1 "P1:"; SParameter2 "P2:"; SParameter3 "P3:"; SParameter4 "P4:"; ShowSpec "表示関数の仕様"
      mask help:
      | このブロックは、以下の Legacy Code Tool の定義で指定されたレガシ関数を呼び出すことができます:
      | def.SFunctionName = 'Motor';
      | def.OutputFcnSpec = 'Motor(double p1, double p2, double p3, double p4, double u1)';
      | def.StartFcnSpec = 'MotorInit()';
      | def.HeaderFiles = {'sfunspikert.h'};
      | def.SourceFiles = {'sfunspikert.c'};
      | def.IncPaths = {'C:\class\coursefiles\SPIKE_Dev\libblocks'};
      mask Help: <p>このブロックは、Legacy Code Tool で自動的に生成されました。このツールと呼び出しの詳細は、ヘルプを参照してください。<a href="matlab:legacy_code('help')"> legacy_code('help')</a>.</p>
      mask Callback ShowSpec:
      | if strcmp(get_param(gcbh, 'ShowSpec'), 'on')
      |   set_param(gcbh, 'MaskDisplay', sprintf('fprintf(''%s'');', get_param(gcbh, 'SFunctionSpec')));
      | else
      |   set_param(gcbh, 'MaskDisplay', sprintf('fprintf(''%s'');', get_param(gcbh, 'FunctionName')));
      | end
      mask Display: fprintf('Motor(double p1, double p2, double p3, double p4, double u1)');
  wires:
  In1/1 -> Motor2/1

== system spikertlib/Powered Up device/PortA Out/Subsystem/None ==
  In1 : Inport
  Terminator : Terminator
  wires:
  In1/1 -> Terminator/1
